simulink model "InverterSignals"  (R2024b)
settings: Solver=FixedStepAuto  StartTime=0.0  StopTime=10.0  RelTol=1e-3
settings Model: DataDictionary=Master_Dictionary.sldd  EnableAccessToBaseWorkspace=off  Creator=torni  LastModifiedBy=will
settings SolverCC: AlgebraicLoopSolver=TrustRegion
settings DataIOCC: ReturnWorkspaceOutputs=off
settings OptimizationCC: DefaultParameterBehavior=Inlined  EnhancedBackFolding=on  PassReuseOutputArgsAs=Individual arguments  ZeroExternalMemoryAtStartup=off  ZeroInternalMemoryAtStartup=off  OptimizeBlockOrder=speed  DifferentSizesBufferReuse=on  OptimizationCustomize=off  EfficientTunableParamExpr=on
settings DebuggingCC: ParameterTunabilityLossMsg=error  UnconnectedInputMsg=warning  UnconnectedOutputMsg=warning  UnconnectedLineMsg=warning  ArithmeticOperatorsInVariantConditions=warning
settings HardwareCC: TargetLargestAtomicInteger=Long  TargetLargestAtomicFloat=Double  TargetIntDivRoundTo=Zero  TargetEndianess=LittleEndian  TargetHWDeviceType=ARM Compatible->ARM Cortex-M  ProdEqTarget=off
settings ModelReferenceCC: EnableRefExpFcnMdlSchedulingChecks=on
settings SFSimCC: MATLABDynamicMemAlloc=off  CustomCodeUndefinedFunction=UseInterfaceOnly
settings RTWCC: Description=Embedded Coder  SystemTargetFile=ert.tlc  TemplateMakefile=ert_default_tmf  Toolchain=GNU Tools for ARM Embedded Processors  RTWCompilerOptimization=on  GPUComputeCapability=3.5
settings CodeAppCC: ForceParamTrailComments=on  IgnoreCustomStorageClasses=off  OperatorAnnotations=on  SimulinkDataObjDesc=on  SFDataObjDesc=on  InsertBlockDesc=on
settings ERTTargetCC: TargetLangStandard=C99 (ISO)  GenerateSampleERTMain=on  ERTCustomFileTemplate=example_file_process.tlc

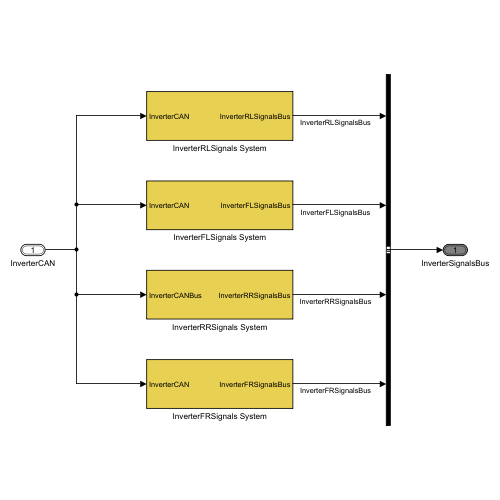
[thumbnail: Simulink's stored preview of the top-level diagram]
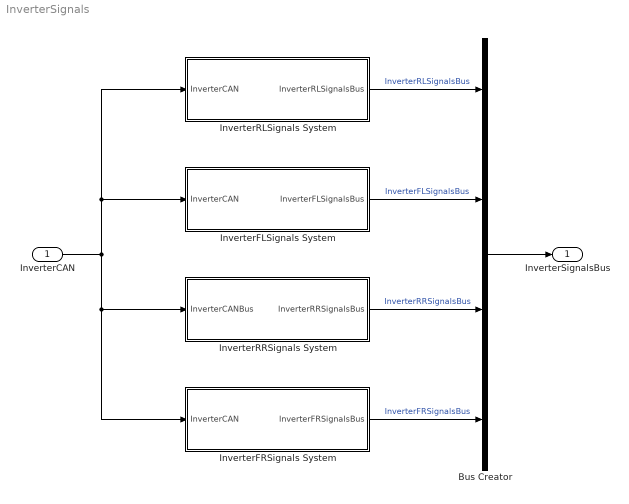
== system InverterSignals ==
  InverterCAN : Inport  OutDataTypeStr=Bus: CAN1_2Bus
  Bus Creator : BusCreator  Inputs=4  OutDataTypeStr=Bus: InverterSignalsBus
  InverterFLSignals System : Subsystem
  InverterFRSignals System : Subsystem
  InverterRLSignals System : Subsystem
  InverterRRSignals System : Subsystem
  InverterSignalsBus : Outport  OutDataTypeStr=Bus: InverterSignalsBus  VectorParamsAs1DForOutWhenUnconnected=off
  wires:
  InverterRLSignals System/1(InverterRLSignalsBus) -> Bus Creator/1  "InverterRLSignalsBus"
  InverterRRSignals System/1(InverterRRSignalsBus) -> Bus Creator/3  "InverterRRSignalsBus"
  InverterFRSignals System/1(InverterFRSignalsBus) -> Bus Creator/4  "InverterFRSignalsBus"
  InverterFLSignals System/1(InverterFLSignalsBus) -> Bus Creator/2  "InverterFLSignalsBus"
  Bus Creator/1 -> InverterSignalsBus/1
  InverterCAN/1 -> InverterFLSignals System/1(InverterCAN), InverterRLSignals System/1(InverterCAN), InverterRRSignals System/1(InverterCANBus), InverterFRSignals System/1(InverterCAN)

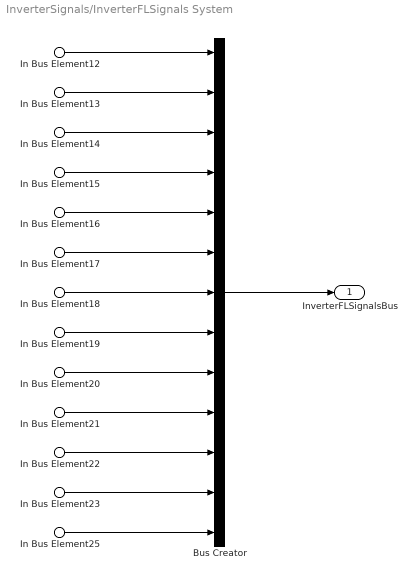
== system InverterSignals/InverterFLSignals System ==
  In Bus Element12 : Inport  PortName=InverterCAN  Element=InverterFLCANBus.nMotorFL
  In Bus Element13 : Inport  PortName=InverterCAN  Element=InverterFLCANBus.BInvDCOnFL
  In Bus Element14 : Inport  PortName=InverterCAN  Element=InverterFLCANBus.BInvErrorFL
  In Bus Element15 : Inport  PortName=InverterCAN  Element=InverterFLCANBus.BInvOnFL
  In Bus Element16 : Inport  PortName=InverterCAN  Element=InverterFLCANBus.BInvDCQuitInvOnFL
  In Bus Element17 : Inport  PortName=InverterCAN  Element=InverterFLCANBus.BInvQuitInvOnFL
  In Bus Element18 : Inport  PortName=InverterCAN  Element=InverterFLCANBus.BInvSysReadyFL
  In Bus Element19 : Inport  PortName=InverterCAN  Element=InverterFLCANBus.BInvWarnFL
  In Bus Element20 : Inport  PortName=InverterCAN  Element=InverterFLCANBus.MMotorMeasuredFL
  In Bus Element21 : Inport  PortName=InverterCAN  Element=InverterFLCANBus.NInvDTCFL
  In Bus Element22 : Inport  PortName=InverterCAN  Element=InverterFLCANBus.TMotorFL
  In Bus Element23 : Inport  PortName=InverterCAN  Element=InverterFLCANBus.VDCInvFL
  In Bus Element25 : Inport  PortName=InverterCAN  Element=InverterFLCANBus.TInvFL
  Bus Creator : BusCreator  Inputs=13  OutDataTypeStr=Bus: InverterFLSignalsBus
  InverterFLSignalsBus : Outport  OutDataTypeStr=Bus: InverterFLSignalsBus  VectorParamsAs1DForOutWhenUnconnected=off
  wires:
  Bus Creator/1 -> InverterFLSignalsBus/1
  In Bus Element12/1 -> Bus Creator/1
  In Bus Element22/1 -> Bus Creator/11
  In Bus Element23/1 -> Bus Creator/12
  In Bus Element25/1 -> Bus Creator/13
  In Bus Element20/1 -> Bus Creator/9
  In Bus Element19/1 -> Bus Creator/8
  In Bus Element18/1 -> Bus Creator/7
  In Bus Element17/1 -> Bus Creator/6
  In Bus Element16/1 -> Bus Creator/5
  In Bus Element15/1 -> Bus Creator/4
  In Bus Element14/1 -> Bus Creator/3
  In Bus Element13/1 -> Bus Creator/2
  In Bus Element21/1 -> Bus Creator/10

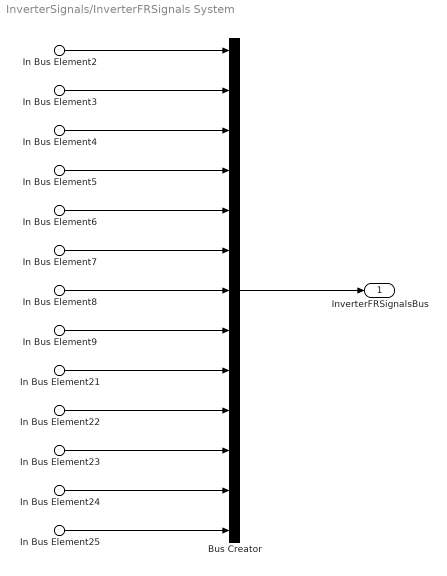
== system InverterSignals/InverterFRSignals System ==
  In Bus Element2 : Inport  PortName=InverterCAN  Element=InverterFRCANBus.nMotorFR
  In Bus Element3 : Inport  PortName=InverterCAN  Element=InverterFRCANBus.BInvDCOnFR
  In Bus Element4 : Inport  PortName=InverterCAN  Element=InverterFRCANBus.BInvErrorFR
  In Bus Element5 : Inport  PortName=InverterCAN  Element=InverterFRCANBus.BInvOnFR
  In Bus Element6 : Inport  PortName=InverterCAN  Element=InverterFRCANBus.BInvDCQuitInvOnFR
  In Bus Element7 : Inport  PortName=InverterCAN  Element=InverterFRCANBus.BInvQuitInvOnFR
  In Bus Element8 : Inport  PortName=InverterCAN  Element=InverterFRCANBus.BInvSysReadyFR
  In Bus Element9 : Inport  PortName=InverterCAN  Element=InverterFRCANBus.BInvWarnFR
  In Bus Element21 : Inport  PortName=InverterCAN  Element=InverterFRCANBus.MMotorMeasuredFR
  In Bus Element22 : Inport  PortName=InverterCAN  Element=InverterFRCANBus.NInvDTCFR
  In Bus Element23 : Inport  PortName=InverterCAN  Element=InverterFRCANBus.TMotorFR
  In Bus Element24 : Inport  PortName=InverterCAN  Element=InverterFRCANBus.VDCInvFR
  In Bus Element25 : Inport  PortName=InverterCAN  Element=InverterFRCANBus.TInvFR
  Bus Creator : BusCreator  Inputs=13  OutDataTypeStr=Bus: InverterFRSignalsBus
  InverterFRSignalsBus : Outport  OutDataTypeStr=Bus: InverterFRSignalsBus  VectorParamsAs1DForOutWhenUnconnected=off
  wires:
  Bus Creator/1 -> InverterFRSignalsBus/1
  In Bus Element2/1 -> Bus Creator/1
  In Bus Element3/1 -> Bus Creator/2
  In Bus Element5/1 -> Bus Creator/4
  In Bus Element6/1 -> Bus Creator/5
  In Bus Element7/1 -> Bus Creator/6
  In Bus Element8/1 -> Bus Creator/7
  In Bus Element9/1 -> Bus Creator/8
  In Bus Element21/1 -> Bus Creator/9
  In Bus Element22/1 -> Bus Creator/10
  In Bus Element23/1 -> Bus Creator/11
  In Bus Element24/1 -> Bus Creator/12
  In Bus Element4/1 -> Bus Creator/3
  In Bus Element25/1 -> Bus Creator/13

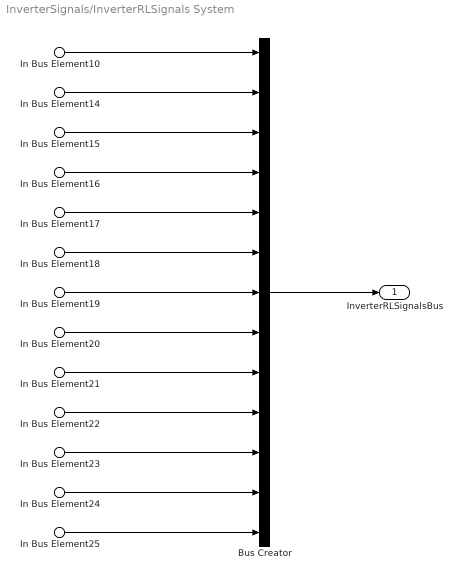
== system InverterSignals/InverterRLSignals System ==
  In Bus Element10 : Inport  PortName=InverterCAN  Element=InverterRLCANBus.nMotorRL
  In Bus Element14 : Inport  PortName=InverterCAN  Element=InverterRLCANBus.BInvDCOnRL
  In Bus Element15 : Inport  PortName=InverterCAN  Element=InverterRLCANBus.BInvErrorRL
  In Bus Element16 : Inport  PortName=InverterCAN  Element=InverterRLCANBus.BInvOnRL
  In Bus Element17 : Inport  PortName=InverterCAN  Element=InverterRLCANBus.BInvDCQuitInvOnRL
  In Bus Element18 : Inport  PortName=InverterCAN  Element=InverterRLCANBus.BInvQuitInvOnRL
  In Bus Element19 : Inport  PortName=InverterCAN  Element=InverterRLCANBus.BInvSysReadyRL
  In Bus Element20 : Inport  PortName=InverterCAN  Element=InverterRLCANBus.BInvWarnRL
  In Bus Element21 : Inport  PortName=InverterCAN  Element=InverterRLCANBus.MMotorMeasuredRL
  In Bus Element22 : Inport  PortName=InverterCAN  Element=InverterRLCANBus.NInvDTCRL
  In Bus Element23 : Inport  PortName=InverterCAN  Element=InverterRLCANBus.TMotorRL
  In Bus Element24 : Inport  PortName=InverterCAN  Element=InverterRLCANBus.VDCInvRL
  In Bus Element25 : Inport  PortName=InverterCAN  Element=InverterRLCANBus.TInvRL
  Bus Creator : BusCreator  Inputs=13  OutDataTypeStr=Bus: InverterRLSignalsBus
  InverterRLSignalsBus : Outport  OutDataTypeStr=Bus: InverterRLSignalsBus  VectorParamsAs1DForOutWhenUnconnected=off
  wires:
  Bus Creator/1 -> InverterRLSignalsBus/1
  In Bus Element10/1 -> Bus Creator/1
  In Bus Element14/1 -> Bus Creator/2
  In Bus Element15/1 -> Bus Creator/3
  In Bus Element16/1 -> Bus Creator/4
  In Bus Element17/1 -> Bus Creator/5
  In Bus Element18/1 -> Bus Creator/6
  In Bus Element19/1 -> Bus Creator/7
  In Bus Element20/1 -> Bus Creator/8
  In Bus Element21/1 -> Bus Creator/9
  In Bus Element23/1 -> Bus Creator/11
  In Bus Element24/1 -> Bus Creator/12
  In Bus Element25/1 -> Bus Creator/13
  In Bus Element22/1 -> Bus Creator/10

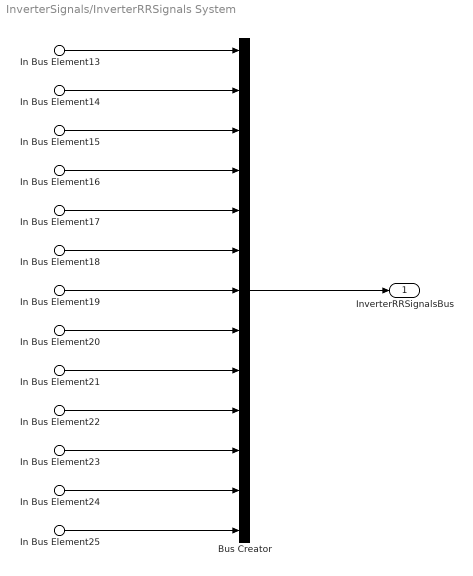
== system InverterSignals/InverterRRSignals System ==
  In Bus Element13 : Inport  PortName=InverterCANBus  Element=InverterRRCANBus.nMotorRR
  In Bus Element14 : Inport  PortName=InverterCANBus  Element=InverterRRCANBus.BInvDCOnRR
  In Bus Element15 : Inport  PortName=InverterCANBus  Element=InverterRRCANBus.BInvErrorRR
  In Bus Element16 : Inport  PortName=InverterCANBus  Element=InverterRRCANBus.BInvOnRR
  In Bus Element17 : Inport  PortName=InverterCANBus  Element=InverterRRCANBus.BInvDCQuitInvOnRR
  In Bus Element18 : Inport  PortName=InverterCANBus  Element=InverterRRCANBus.BInvQuitInvOnRR
  In Bus Element19 : Inport  PortName=InverterCANBus  Element=InverterRRCANBus.BInvSysReadyRR
  In Bus Element20 : Inport  PortName=InverterCANBus  Element=InverterRRCANBus.BInvWarnRR
  In Bus Element21 : Inport  PortName=InverterCANBus  Element=InverterRRCANBus.MMotorMeasuredRR
  In Bus Element22 : Inport  PortName=InverterCANBus  Element=InverterRRCANBus.NInvDTCRR
  In Bus Element23 : Inport  PortName=InverterCANBus  Element=InverterRRCANBus.TMotorRR
  In Bus Element24 : Inport  PortName=InverterCANBus  Element=InverterRRCANBus.VDCInvRR
  In Bus Element25 : Inport  PortName=InverterCANBus  Element=InverterRRCANBus.TInvRR
  Bus Creator : BusCreator  Inputs=13  OutDataTypeStr=Bus: InverterRRSignalsBus
  InverterRRSignalsBus : Outport  OutDataTypeStr=Bus: InverterRRSignalsBus  VectorParamsAs1DForOutWhenUnconnected=off
  wires:
  Bus Creator/1 -> InverterRRSignalsBus/1
  In Bus Element13/1 -> Bus Creator/1
  In Bus Element14/1 -> Bus Creator/2
  In Bus Element15/1 -> Bus Creator/3
  In Bus Element16/1 -> Bus Creator/4
  In Bus Element17/1 -> Bus Creator/5
  In Bus Element18/1 -> Bus Creator/6
  In Bus Element19/1 -> Bus Creator/7
  In Bus Element20/1 -> Bus Creator/8
  In Bus Element21/1 -> Bus Creator/9
  In Bus Element22/1 -> Bus Creator/10
  In Bus Element23/1 -> Bus Creator/11
  In Bus Element24/1 -> Bus Creator/12
  In Bus Element25/1 -> Bus Creator/13
